simulink library "sm_cam_flapping_wing_lib"  (R2021b)
settings: Solver=ode45  StartTime=0.0  StopTime=10.0  RelTol=1e-3  EnableMultiTasking=on
undefined symbols (not defined in the file): colors, rhos, X, Y, Z
libraries: sm_lib x8
settings Model: Creator=The MathWorks, Inc.  LastModifiedBy=The MathWorks, Inc.
settings SolverCC: AlgebraicLoopSolver=TrustRegion
settings DataIOCC: LimitDataPoints=on  ReturnWorkspaceOutputs=off
settings OptimizationCC: LifeSpan=inf
settings DebuggingCC: AllowSymbolicDim=off  SFUnexpectedBacktrackingDiag=warning  SFNoUnconditionalDefaultTransitionDiag=warning  SFExecutionAtInitializationDiag=none  SFMachineParentedDataDiag=warning  ArithmeticOperatorsInVariantConditions=warning
settings HardwareCC: ProdBitPerPointer=32  ProdBitPerSizeT=32  ProdBitPerPtrDiffT=32  ProdLargestAtomicFloat=None  ProdIntDivRoundTo=Undefined  ProdEndianess=Unspecified  ProdWordSize=32  ProdHWDeviceType=32-bit Generic
settings ModelReferenceCC: PropagateSignalLabelsOutOfModel=off
settings SFSimCC: SimUseLocalCustomCode=off  CustomCodeUndefinedFunction=UseInterfaceOnly
settings RTWCC: RTWUseLocalCustomCode=off
settings CodeAppCC: StateflowObjectComments=on
settings GRTTargetCC: TargetLangStandard=C89/C90 (ANSI)
settings ConfigComp: CovMetricSettings=dw  CovSaveCumulativeToWorkspaceVar=on  CovSaveSingleToWorkspaceVar=on  CovExternalEMLEnable=off

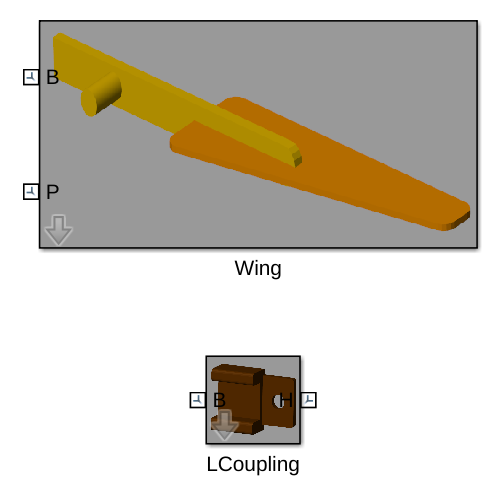
[thumbnail: Simulink's stored preview of the top-level diagram]
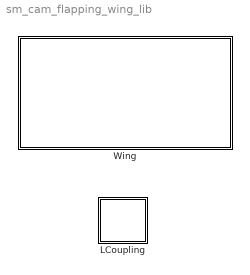
== system sm_cam_flapping_wing_lib ==
  LCoupling : Subsystem  mask(Left Coupling){H=5, W=2.5, L=7, Hs=3, Ws=1.5, Ls=4, Rh=0.6, Tf=0.5, Rc=0.25, rho=rhos.aluminum, col=colors.brown}
      mask prompts: H "H - Height (cm):"; W "W - Width (cm):"; L "L - Length (cm):"; Hs "Hs - Slot height (cm):"; Ws "Ws - Slot width (cm):"; Ls "Ls - Slot length (cm):"; Rh "Rh - Hole radius (cm):"; Tf "Tf - Flange thickness (cm):"; Rc "Rc - Chamfer radius (cm):"; rho "Density (kg/m^3):"; col "Color [R G B]:"
      mask help:
      | Coupling that connects the left wing to the right wing. The coupling slides on the wing link.
      |
      | Click on the help button for parameter information.
      mask init:
      | slot_xsec = [-Ws/2 Hs/2; Ws/2 Hs/2; Ws/2 H/2; -W+Ws/2 H/2; ...
      |              -W+Ws/2 -H/2; Ws/2 -H/2; Ws/2 -Hs/2; -Ws/2 -Hs/2];
      |          
      | slot_xsec = simmechanics.demohelpers.round_corners(slot_xsec, [2 3 4 5 6 7], Rc, 5);
      | 
      | Hf = 0.8*H;
      | flange_xsec = [(L-Ls)/2 0; (L-Ls)/2 Hf/2; -(L-Ls)/2 Hf/2; ...
      |               -(L-Ls)/2 -Hf/2; (L-Ls)/2 -Hf/2; (L-Ls)/2 0];
      | 
      | flange_xsec = simmechanics.demohelpers.round_corners(flange_xsec, ...
      |                 [3 4], Rc, 5);          
      |           
      | th = (0:-10:-360)'*pi/180;          
      | hole_xsec = [Rh*cos(th) Rh*sin(th)];
      | 
      | flange_xsec = [flange_xsec; hole_xsec];
      mask Help: web(['file:///' fullfile(matlabroot,'toolbox','physmod','sm','smdemos','cam_flapping_wing','images','sm_camflappingwing_lcoupling_dims.svg')],'-notoolbar','-new')
      mask DialogControl Container4 Prompt: Dimensions
      mask DialogControl Container5 Prompt: Material Properties
      mask Display:
      | image(fullfile(matlabroot,'toolbox','physmod','sm','smdemos','cam_flapping_wing','images','sm_camflappingwing_lcoupling.png'));
      | port_label('Lconn',1,'B');
      | port_label('Rconn',1,'H');
  Wing : Subsystem  mask(Flapping Wing){W=1, T=3, L=30, Dp=7.5, Lp=4, Rp=1, Rc=1.25, Ow=10, Wwb=10, Wwt=4, Lw=30, Tw=0.5, rho=2700, lclr=[1 0.8 0], wclr=[1 0.6 0]}
      mask prompts: W "W - Link Width (cm):"; T "T - Link Thickness (cm):"; L "L - Link Length (cm):"; Dp "Dp - Peg distance (cm):"; Lp "Lp - Peg legth (cm):"; Rp "Rp - Peg Radius (cm):"; Rc "Rc - Chamfer radius (cm):"; Ow "Ow - Wing offset (cm):"; Wwb "Wwb - Wing base width (cm):"; Wwt "Wwt - Wing tip width (cm):"; Lw "Lw - Wing length (cm):"; Tw "Tw - Wing thickness (cm):"; rho "Density (kg/m^3):"; lclr "Link Color [R G B]:"; wclr "Wing Color [R G B]:"
      mask help: Click on the help button for parameter information.
      mask init:
      | link_xsec = [-Dp -T/2; L-Dp -T/2; L-Dp T/2; -Dp T/2];
      | link_xsec = simmechanics.demohelpers.round_corners(link_xsec,[2 3], Rc, 5);
      | 
      | 
      | 
      | wing_xsec = [0 -Wwb/4; 0 -Wwb/2; Lw -Wwb/2; Lw (Wwt-Wwb/2); 0 Wwb/2; 0 Wwb/4];
      | wing_xsec = simmechanics.demohelpers.round_corners(wing_xsec,[2 3 4 5], Rc, 5);
      mask Help: web(['file:///' fullfile(matlabroot,'toolbox','physmod','sm','smdemos','cam_flapping_wing','images','sm_camflappingwing_wing_dims.svg')],'-notoolbar','-new')
      mask DialogControl Container4 Prompt: Dimensions
      mask DialogControl Container6 Prompt: Wing
      mask DialogControl Container5 Prompt: Material Properties
      mask Display:
      | image(fullfile(matlabroot,'toolbox','physmod','sm','smdemos','cam_flapping_wing','images','sm_camflappingwing_wing.png'));
      | port_label('Lconn',1,'B');
      | port_label('Lconn',2,'P');

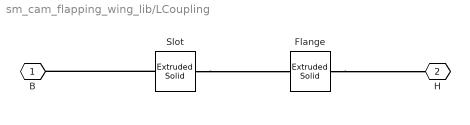
== system sm_cam_flapping_wing_lib/LCoupling ==
  Flange : sm_lib/Body Elements/Extruded Solid  GraphicAmbientColor=[0.15 0.15 0.15 1.0]  BasedOnType=Density  CenterOfMass=[0 0 0]  CenterOfMassUnits=m  GraphicDiffuseColor=col  ExportConvexHullGeometry=off  ExtrusionCrossSection=flange_xsec  ExtrusionCrossSectionUnits=cm  Density=rho  DensityUnits=kg/(m^3)  DoExposeReferenceFrame=on  GraphicEmissiveColor=[0.0 0.0 0.0 1.0]  ExportEntireGeometry=off  ExtrusionLength=Tf  ExtrusionLengthUnits=cm  ExtrusionType=General  SerializedFrames=<Frames><Frame><Id>Frame1</Id><Value><Name>B</Name><Origin><Source>GeometricFeature</Source><FeatureName>bottom point 1</FeatureName></Origin><PrimaryAxis><DefinedDirection>-Z</DefinedDirection><Source>ReferenceFrame</Source><SourceDirection>+X</SourceDirection><FeatureName></FeatureName></PrimaryAxis><SecondaryAxis><DefinedDirection>+X</DefinedDirection><Source>ReferenceFrame</Source><SourceDirection>+Z</SourceDirection><FeatureName></FeatureName></SecondaryAxis></Value></Frame></Frames>  MarkerShape=Sphere  MarkerSize=10  GraphicType=FromGeometry  InertiaType=CalculateFromGeometry  Mass=1  MassUnits=kg  MomentsOfInertia=[1 1 1]  MomentsOfInertiaUnits=kg*m^2  PolygonNumSides=3  GraphicOpacity=1.0  PolygonOuterRadius=1  PolygonOuterRadiusUnits=m  ProductsOfInertia=[0 0 0]  ProductsOfInertiaUnits=kg*m^2  GraphicShininess=75  GraphicSpecularColor=[0.5 0.5 0.5 1.0]  GraphicVisPropType=SimpleVisualProperties
  Slot : sm_lib/Body Elements/Extruded Solid  GraphicAmbientColor=[0.15 0.15 0.15 1.0]  BasedOnType=Density  CenterOfMass=[0 0 0]  CenterOfMassUnits=m  GraphicDiffuseColor=col  ExportConvexHullGeometry=off  ExtrusionCrossSection=slot_xsec  ExtrusionCrossSectionUnits=cm  Density=rho  DensityUnits=kg/(m^3)  DoExposeReferenceFrame=on  GraphicEmissiveColor=[0.0 0.0 0.0 1.0]  ExportEntireGeometry=off  ExtrusionLength=Ls  ExtrusionLengthUnits=cm  ExtrusionType=General  SerializedFrames=<Frames><Frame><Id>Frame1</Id><Value><Name>T</Name><Origin><Source>GeometricFeature</Source><FeatureName>top curve 16</FeatureName></Origin><PrimaryAxis><DefinedDirection>+Z</DefinedDirection><Source>ReferenceFrame</Source><SourceDirection>+Z</SourceDirection><FeatureName></FeatureName></PrimaryAxis><SecondaryAxis><DefinedDirection>+X</DefinedDirection><Source>ReferenceFrame</Source><SourceDirection>+X</SourceDirection><FeatureName></FeatureName></SecondaryAxis></Value></Frame></Frames>  MarkerShape=Sphere  MarkerSize=10  GraphicType=FromGeometry  InertiaType=CalculateFromGeometry  Mass=1  MassUnits=kg  MomentsOfInertia=[1 1 1]  MomentsOfInertiaUnits=kg*m^2  PolygonNumSides=3  GraphicOpacity=1.0  PolygonOuterRadius=1  PolygonOuterRadiusUnits=m  ProductsOfInertia=[0 0 0]  ProductsOfInertiaUnits=kg*m^2  GraphicShininess=75  GraphicSpecularColor=[0.5 0.5 0.5 1.0]  GraphicVisPropType=SimpleVisualProperties
  B : PMIOPort  Side=Left
  H : PMIOPort  Port=2  Side=Right
  connections:
  Flange/RConn1 -- H/RConn1
  Slot/LConn1 -- Flange/LConn1
  Slot/RConn1 -- B/RConn1

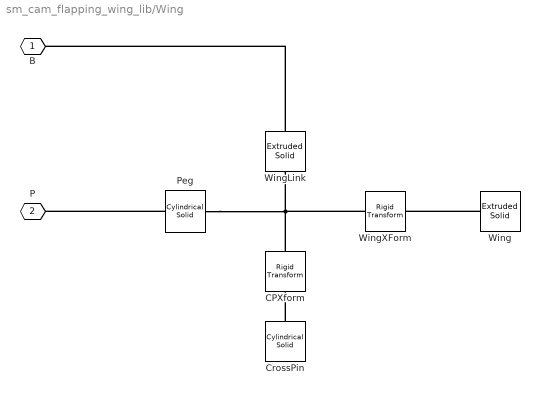
== system sm_cam_flapping_wing_lib/Wing ==
  CPXform : sm_lib/Frames and Transforms/Rigid Transform  TranslationMethod=StandardAxis  TranslationStandardOffset=3*Lp/4  TranslationLengthUnit=cm  TranslationStandardAxis=+Z  TranslationCartesianOffset=[0 0 0]  TranslationROffset=0  TranslationROffsetUnits=m  TranslationZOffset=0  TranslationZOffsetUnits=m  TranslationThetaOffset=0  TranslationThetaOffsetUnits=deg  RotationMethod=AlignedAxes  RotationAngleUnits=deg  RotationStandardAxis=+Z  RotationAngle=0.0  RotationArbitraryAxis=[0 0 1]  FollAlignAxisA=+Z  BaseAlignAxisA=+Y  FollAlignAxisB=+Y  BaseAlignAxisB=-Z  RotationSequenceAxes=FollowerAxes  RotationSequence=XYX  RotationSequenceAngles=[0 0 0]  RotationSequenceAnglesUnits=deg  RotationMatrix=[1 0 0; 0 1 0; 0 0 1]
  CrossPin : sm_lib/Body Elements/Cylindrical Solid  GraphicAmbientColor=[0.15 0.15 0.15 1.0]  BasedOnType=Density  CenterOfMass=[0 0 0]  CenterOfMassUnits=m  GraphicDiffuseColor=lclr  CylinderLength=3*Rp  CylinderLengthUnits=cm  CylinderRadius=Rp/2  CylinderRadiusUnits=cm  Density=rho  DensityUnits=kg/(m^3)  DoExposeReferenceFrame=on  GraphicEmissiveColor=[0.0 0.0 0.0 1.0]  ExportEntireGeometry=off  SerializedFrames=<Frames/>  MarkerShape=Sphere  MarkerSize=10  GraphicType=FromGeometry  InertiaType=CalculateFromGeometry  Mass=1  MassUnits=kg  MomentsOfInertia=[1 1 1]  MomentsOfInertiaUnits=kg*m^2  GraphicOpacity=1.0  ProductsOfInertia=[0 0 0]  ProductsOfInertiaUnits=kg*m^2  GraphicShininess=75  GraphicSpecularColor=[0.5 0.5 0.5 1.0]  GraphicVisPropType=SimpleVisualProperties
  Peg : sm_lib/Body Elements/Cylindrical Solid  GraphicAmbientColor=[0.15 0.15 0.15 1.0]  BasedOnType=Density  CenterOfMass=[0 0 0]  CenterOfMassUnits=m  GraphicDiffuseColor=lclr  CylinderLength=Lp  CylinderLengthUnits=cm  CylinderRadius=Rp  CylinderRadiusUnits=cm  Density=rho  DensityUnits=kg/(m^3)  DoExposeReferenceFrame=on  GraphicEmissiveColor=[0.0 0.0 0.0 1.0]  ExportEntireGeometry=off  SerializedFrames=<Frames><Frame><Id>Frame2</Id><Value><Name>B</Name><Origin><Source>GeometricFeature</Source><FeatureName>bottom surface</FeatureName></Origin><PrimaryAxis><DefinedDirection>+Z</DefinedDirection><Source>ReferenceFrame</Source><SourceDirection>+Z</SourceDirection><FeatureName></FeatureName></PrimaryAxis><SecondaryAxis><DefinedDirection>+X</DefinedDirection><Source>ReferenceFrame</Source><SourceDirection>+X</SourceDirection><FeatureName></FeatureName></SecondaryAxis></Value></Frame></Frames>  MarkerShape=Sphere  MarkerSize=10  GraphicType=FromGeometry  InertiaType=CalculateFromGeometry  Mass=1  MassUnits=kg  MomentsOfInertia=[1 1 1]  MomentsOfInertiaUnits=kg*m^2  GraphicOpacity=1.0  ProductsOfInertia=[0 0 0]  ProductsOfInertiaUnits=kg*m^2  GraphicShininess=75  GraphicSpecularColor=[0.5 0.5 0.5 1.0]  GraphicVisPropType=SimpleVisualProperties
  Wing : sm_lib/Body Elements/Extruded Solid  GraphicAmbientColor=[0.15 0.15 0.15 1.0]  BasedOnType=Density  CenterOfMass=[0 0 0]  CenterOfMassUnits=m  GraphicDiffuseColor=wclr  ExportConvexHullGeometry=off  ExtrusionCrossSection=wing_xsec  ExtrusionCrossSectionUnits=cm  Density=rho  DensityUnits=kg/(m^3)  DoExposeReferenceFrame=on  GraphicEmissiveColor=[0.0 0.0 0.0 1.0]  ExportEntireGeometry=off  ExtrusionLength=Tw  ExtrusionLengthUnits=cm  ExtrusionType=General  SerializedFrames=<Frames/>  MarkerShape=Sphere  MarkerSize=10  GraphicType=FromGeometry  InertiaType=CalculateFromGeometry  Mass=1  MassUnits=kg  MomentsOfInertia=[1 1 1]  MomentsOfInertiaUnits=kg*m^2  PolygonNumSides=3  GraphicOpacity=1.0  PolygonOuterRadius=1  PolygonOuterRadiusUnits=m  ProductsOfInertia=[0 0 0]  ProductsOfInertiaUnits=kg*m^2  GraphicShininess=75  GraphicSpecularColor=[0.5 0.5 0.5 1.0]  GraphicVisPropType=SimpleVisualProperties
  WingLink : sm_lib/Body Elements/Extruded Solid  GraphicAmbientColor=[0.15 0.15 0.15 1.0]  BasedOnType=Density  CenterOfMass=[0 0 0]  CenterOfMassUnits=m  GraphicDiffuseColor=lclr  ExportConvexHullGeometry=off  ExtrusionCrossSection=link_xsec  ExtrusionCrossSectionUnits=cm  Density=rho  DensityUnits=kg/(m^3)  DoExposeReferenceFrame=on  GraphicEmissiveColor=[0.0 0.0 0.0 1.0]  ExportEntireGeometry=off  ExtrusionLength=W  ExtrusionLengthUnits=cm  ExtrusionType=General  SerializedFrames=<Frames><Frame><Id>Frame1</Id><Value><Name>B</Name><Origin><Source>GeometricFeature</Source><FeatureName>side surface 12</FeatureName></Origin><PrimaryAxis><DefinedDirection>-Z</DefinedDirection><Source>ReferenceFrame</Source><SourceDirection>+X</SourceDirection><FeatureName></FeatureName></PrimaryAxis><SecondaryAxis><DefinedDirection>+Y</DefinedDirection><Source>ReferenceFrame</Source><SourceDirection>+Y</SourceDirection><FeatureName></FeatureName></SecondaryAxis></Value></Frame></Frames>  MarkerShape=Sphere  MarkerSize=10  GraphicType=FromGeometry  InertiaType=CalculateFromGeometry  Mass=1  MassUnits=kg  MomentsOfInertia=[1 1 1]  MomentsOfInertiaUnits=kg*m^2  PolygonNumSides=3  GraphicOpacity=1.0  PolygonOuterRadius=1  PolygonOuterRadiusUnits=m  ProductsOfInertia=[0 0 0]  ProductsOfInertiaUnits=kg*m^2  GraphicShininess=75  GraphicSpecularColor=[0.5 0.5 0.5 1.0]  GraphicVisPropType=SimpleVisualProperties
  WingXForm : sm_lib/Frames and Transforms/Rigid Transform  TranslationMethod=StandardAxis  TranslationStandardOffset=Ow  TranslationLengthUnit=cm  TranslationStandardAxis=+X  TranslationCartesianOffset=[0 0 0]  TranslationROffset=0  TranslationROffsetUnits=m  TranslationZOffset=0  TranslationZOffsetUnits=m  TranslationThetaOffset=0  TranslationThetaOffsetUnits=deg  RotationMethod=AlignedAxes  RotationAngleUnits=deg  RotationStandardAxis=+Z  RotationAngle=0.0  RotationArbitraryAxis=[0 0 1]  FollAlignAxisA=+Y  BaseAlignAxisA=+Z  FollAlignAxisB=+X  BaseAlignAxisB=+X  RotationSequenceAxes=FollowerAxes  RotationSequence=XYX  RotationSequenceAngles=[0 0 0]  RotationSequenceAnglesUnits=deg  RotationMatrix=[1 0 0; 0 1 0; 0 0 1]
  B : PMIOPort  Side=Left
  P : PMIOPort  Port=2  Side=Left
  connections:
  WingLink/LConn1 -- B/RConn1
  Peg/LConn1 -- WingXForm/LConn1 -- CPXform/LConn1 -- WingLink/RConn1
  Peg/RConn1 -- P/RConn1
  Wing/RConn1 -- WingXForm/RConn1
  CrossPin/RConn1 -- CPXform/RConn1
